simulink model "FullEKF_2007a"  (Simulink 6.6)
settings: Solver=FixedStepDiscrete  StartTime=0.0  StopTime=300  FixedStep=0.01  RelTol=1e-3
values from neighbouring files (symbols this model uses):
  initP = diag([1e-3 1e-3 1e-3 1e-6 1e-6 1e-6 1 1 1 5e-6 5e-6 5e-6 1e-8 1e-8 1e-8])    [FullEKF_init.m.m]
undefined symbols (not defined in the file or in its folder): DiscIntNeverNeededParam, gcbh, hwbcalib_subsystem
libraries: simulink x6, dspmtrx3 x4, dspinverses x1
(part 6 of 7)

== system FullEKF_2007a/INS/Attitude update/Stage2/Subsystem/a23 ==
  quat : Inport  OutDataType=fixdt(1,16,0)  OutScaling=[]  Interpolate=off  mask(Inport (HW)){maskPort=1, PortWidth=0, BusOuputAsStruct=0, signalName=<, Unit=, lowerRange=, upperRange=, InitOut=, latch=Latched}
      mask prompts: maskPort "Mask Port"; PortWidth "Dimensions (-1 for dynamic):"; BusOuputAsStruct "Output as Non-Virtual:"; signalName "Signal Name"; lowerRange "Lower Range"; upperRange "Upper Range"; InitOut "Software Initial Output"; latch "DEOS Consumed Type"
      mask init:
      | %hwbcalib_inport(gcbh,'done');
      settings: CopyFcn=hwbcalib_copyfcn(gcbh);  UndoDeleteFcn=hwbcalib_inport(gcbh,'undodelete');  ModelCloseFcn=set_param(gcbh,'DeleteFcn','');  OpenFcn=hwbcalib_inport(gcbh,0);  PreDeleteFcn=hwbcalib_inport(gcbh,'delete');
      mask Help: file:///../../../Inport.html
      mask StyleString: edit,edit,edit,edit,edit,edit,edit,edit,popup(Latched|Not Latched)
      mask Display:
      | text(4,8,['quat   [' maskPort ']'],'Horizontal','left','Vertical','middle')
      | plot([0 50-10],[0 0]);
      | plot([0 0],[0 16]);
      | plot([0 50-10],[16 16]);
      | plot([50-10 50],[16 8]);
      | plot([50-10 50],[0 8]);
  BorderBottom : Subsystem
      settings: AttributesFormatString="* HONEYWELL PROPRIETARY AND CONFIDENTIAL * Copyright (c) 1996-2011 Honeywell International Inc. * Unpublished Work.  All rights reserved. *"
      mask Type: Border (HW)
      mask Description: Border
  BorderLeft : Subsystem
      mask Type: Border (HW)
      mask Description: Border
  BorderRight : Subsystem
      mask Type: Border (HW)
      mask Description: Border
  BorderTop : Subsystem
      mask Type: Border (HW)
      mask Description: Border
  Subsystem Revision : Subsystem  mask(Subsystem Revision (HW)){trace=}
      mask prompts: trace "Trace Tag:"
      settings: CopyFcn=hwbcalib_copyfcn(gcbh);  OpenFcn=hwbcalib_subrevision(gcbh,0);
      mask Help: file:///../../../Subsystem_Revision.html
      mask Display: disp('Program: \nCPU/Process: /D:\nDLL: tgen\nFilename: INS_ham_napokusy.mdl\nSubsystem: INS/Attitude update/Stage1/quatToDcm/a23\n\nHAM Library Version: 6.5.0\nRevision: -\nDate: 07-Dec-2011 at 09:52:57\nModel Update Rate: 100 Hz\n[ode3]\nTrace Tag: \n\nPage: 18 of 53, Parent Page: 12')
  deMux : Subsystem  mask(Demux (HW)){num=4}
      mask prompts: num "Number of Outputs"
      mask init:
      | %hwbcalib_doDoneCallback('hwbcalib_demux',gcbh,99);
      settings: CopyFcn=hwbcalib_copyfcn(gcbh);  OpenFcn=hwbcalib_demux(gcbh,0);
      mask Help: file:///../../../De-Multiplexer.html
  gain : Subsystem  mask(Gain (HW)){gain=2, Ts=1/100}
      mask prompts: Ts "Sample Time"
      mask init:
      | %hwbcalib_doDoneCallback('hwbcalib_gain',gcbh,99);
      settings: CopyFcn=hwbcalib_copyfcn(gcbh);  OpenFcn=hwbcalib_gain(gcbh,0);
      mask Help: file:///../../../Gain.html
      mask Display: disp('k=2')
  product : Subsystem  mask(Product (HW)){num=2}
      mask prompts: num "Numer of Inputs"
      mask init:
      | %hwbcalib_doDoneCallback('hwbcalib_product',gcbh,99);
      settings: CopyFcn=hwbcalib_copyfcn(gcbh);  OpenFcn=hwbcalib_product(gcbh,0);
      mask Help: file:///../../../Product.html
      mask Display: disp('X')
  product1 : Subsystem  mask(Product (HW)){num=2}
      mask prompts: num "Numer of Inputs"
      mask init:
      | %hwbcalib_doDoneCallback('hwbcalib_product',gcbh,99);
      settings: CopyFcn=hwbcalib_copyfcn(gcbh);  OpenFcn=hwbcalib_product(gcbh,0);
      mask Help: file:///../../../Product.html
      mask Display: disp('X')
  sum : Subsystem  mask(Sum (HW)){signs=++}
      mask prompts: signs "String of Signs"
      mask init:
      | %hwbcalib_doDoneCallback('hwbcalib_sum',gcbh,99);
      settings: CopyFcn=hwbcalib_copyfcn(gcbh);  OpenFcn=hwbcalib_sum(gcbh,0);
      mask Help: file:///../../../Summation.html
      mask Display:
      | text(0.2, (20*(2-1)+11)/40, '+');
      | text(0.2, (20*(1-1)+11)/40, '+');
  a23 : Outport  OutDataType=fixdt(1,16,0)  OutScaling=[]  mask(Outport (HW)){maskPort=1, PortWidth=0, lowerRange=, upperRange=, signalName=<, Unit=}
      mask prompts: maskPort "Mask Port"; PortWidth "Dimensions (-1 for dynamic):"; lowerRange "Lower Range"; upperRange "Upper Range"; signalName "Signal Name"; Unit "Units"
      mask init:
      | %hwbcalib_outport(gcbh,'done');
      settings: CopyFcn=hwbcalib_copyfcn(gcbh);  UndoDeleteFcn=hwbcalib_outport(gcbh,'undodelete');  ModelCloseFcn=set_param(gcbh,'DeleteFcn','');  OpenFcn=hwbcalib_outport(gcbh,0);  PreDeleteFcn=hwbcalib_outport(gcbh,'delete');
      mask Help: file:///../../../Outport.html
      mask Display:
      | text(50-4,8,['a23   [' maskPort ']'],'Horizontal','right','Vertical','middle')
      | plot([10 50],[0 0]);
      | plot([50-1 50-1],[0 16]);
      | plot([10 50],[16 16]);
      | plot([0 10],[8 16]);
      | plot([0 10],[8 0]);
  wires:
  quat/1 -> deMux/1(Dmx)
  product/1(1000) -> sum/1(1)
  product1/1(1000) -> sum/2(2)
  sum/1(1000) -> gain/1(1)
  gain/1(2) -> a23/1
  deMux/1(1) -> product/1(1)
  deMux/2(2) -> product/2(2)
  deMux/3(3) -> product1/1(1)
  deMux/4(4) -> product1/2(2)

== system FullEKF_2007a/INS/Attitude update/Stage2/Subsystem/a31 ==
  quat : Inport  OutDataType=fixdt(1,16,0)  OutScaling=[]  Interpolate=off  mask(Inport (HW)){maskPort=1, PortWidth=0, BusOuputAsStruct=0, signalName=<, Unit=, lowerRange=, upperRange=, InitOut=, latch=Latched}
      mask prompts: maskPort "Mask Port"; PortWidth "Dimensions (-1 for dynamic):"; BusOuputAsStruct "Output as Non-Virtual:"; signalName "Signal Name"; lowerRange "Lower Range"; upperRange "Upper Range"; InitOut "Software Initial Output"; latch "DEOS Consumed Type"
      mask init:
      | %hwbcalib_inport(gcbh,'done');
      settings: CopyFcn=hwbcalib_copyfcn(gcbh);  UndoDeleteFcn=hwbcalib_inport(gcbh,'undodelete');  ModelCloseFcn=set_param(gcbh,'DeleteFcn','');  OpenFcn=hwbcalib_inport(gcbh,0);  PreDeleteFcn=hwbcalib_inport(gcbh,'delete');
      mask Help: file:///../../../Inport.html
      mask StyleString: edit,edit,edit,edit,edit,edit,edit,edit,popup(Latched|Not Latched)
      mask Display:
      | text(4,8,['quat   [' maskPort ']'],'Horizontal','left','Vertical','middle')
      | plot([0 50-10],[0 0]);
      | plot([0 0],[0 16]);
      | plot([0 50-10],[16 16]);
      | plot([50-10 50],[16 8]);
      | plot([50-10 50],[0 8]);
  BorderBottom : Subsystem
      settings: AttributesFormatString="* HONEYWELL PROPRIETARY AND CONFIDENTIAL * Copyright (c) 1996-2011 Honeywell International Inc. * Unpublished Work.  All rights reserved. *"
      mask Type: Border (HW)
      mask Description: Border
  BorderLeft : Subsystem
      mask Type: Border (HW)
      mask Description: Border
  BorderRight : Subsystem
      mask Type: Border (HW)
      mask Description: Border
  BorderTop : Subsystem
      mask Type: Border (HW)
      mask Description: Border
  Subsystem Revision : Subsystem  mask(Subsystem Revision (HW)){trace=}
      mask prompts: trace "Trace Tag:"
      settings: CopyFcn=hwbcalib_copyfcn(gcbh);  OpenFcn=hwbcalib_subrevision(gcbh,0);
      mask Help: file:///../../../Subsystem_Revision.html
      mask Display: disp('Program: \nCPU/Process: /D:\nDLL: tgen\nFilename: INS_ham_napokusy.mdl\nSubsystem: INS/Attitude update/Stage1/quatToDcm/a31\n\nHAM Library Version: 6.5.0\nRevision: -\nDate: 07-Dec-2011 at 09:52:57\nModel Update Rate: 100 Hz\n[ode3]\nTrace Tag: \n\nPage: 19 of 53, Parent Page: 12')
  deMux : Subsystem  mask(Demux (HW)){num=4}
      mask prompts: num "Number of Outputs"
      mask init:
      | %hwbcalib_doDoneCallback('hwbcalib_demux',gcbh,99);
      settings: CopyFcn=hwbcalib_copyfcn(gcbh);  OpenFcn=hwbcalib_demux(gcbh,0);
      mask Help: file:///../../../De-Multiplexer.html
  gain : Subsystem  mask(Gain (HW)){gain=2, Ts=1/100}
      mask prompts: Ts "Sample Time"
      mask init:
      | %hwbcalib_doDoneCallback('hwbcalib_gain',gcbh,99);
      settings: CopyFcn=hwbcalib_copyfcn(gcbh);  OpenFcn=hwbcalib_gain(gcbh,0);
      mask Help: file:///../../../Gain.html
      mask Display: disp('k=2')
  product : Subsystem  mask(Product (HW)){num=2}
      mask prompts: num "Numer of Inputs"
      mask init:
      | %hwbcalib_doDoneCallback('hwbcalib_product',gcbh,99);
      settings: CopyFcn=hwbcalib_copyfcn(gcbh);  OpenFcn=hwbcalib_product(gcbh,0);
      mask Help: file:///../../../Product.html
      mask Display: disp('X')
  product1 : Subsystem  mask(Product (HW)){num=2}
      mask prompts: num "Numer of Inputs"
      mask init:
      | %hwbcalib_doDoneCallback('hwbcalib_product',gcbh,99);
      settings: CopyFcn=hwbcalib_copyfcn(gcbh);  OpenFcn=hwbcalib_product(gcbh,0);
      mask Help: file:///../../../Product.html
      mask Display: disp('X')
  sum : Subsystem  mask(Sum (HW)){signs=++}
      mask prompts: signs "String of Signs"
      mask init:
      | %hwbcalib_doDoneCallback('hwbcalib_sum',gcbh,99);
      settings: CopyFcn=hwbcalib_copyfcn(gcbh);  OpenFcn=hwbcalib_sum(gcbh,0);
      mask Help: file:///../../../Summation.html
      mask Display:
      | text(0.2, (20*(2-1)+11)/40, '+');
      | text(0.2, (20*(1-1)+11)/40, '+');
  a31 : Outport  OutDataType=fixdt(1,16,0)  OutScaling=[]  mask(Outport (HW)){maskPort=1, PortWidth=0, lowerRange=, upperRange=, signalName=<, Unit=}
      mask prompts: maskPort "Mask Port"; PortWidth "Dimensions (-1 for dynamic):"; lowerRange "Lower Range"; upperRange "Upper Range"; signalName "Signal Name"; Unit "Units"
      mask init:
      | %hwbcalib_outport(gcbh,'done');
      settings: CopyFcn=hwbcalib_copyfcn(gcbh);  UndoDeleteFcn=hwbcalib_outport(gcbh,'undodelete');  ModelCloseFcn=set_param(gcbh,'DeleteFcn','');  OpenFcn=hwbcalib_outport(gcbh,0);  PreDeleteFcn=hwbcalib_outport(gcbh,'delete');
      mask Help: file:///../../../Outport.html
      mask Display:
      | text(50-4,8,['a31   [' maskPort ']'],'Horizontal','right','Vertical','middle')
      | plot([10 50],[0 0]);
      | plot([50-1 50-1],[0 16]);
      | plot([10 50],[16 16]);
      | plot([0 10],[8 16]);
      | plot([0 10],[8 0]);
  wires:
  quat/1 -> deMux/1(Dmx)
  product/1(1000) -> sum/1(1)
  product1/1(1000) -> sum/2(2)
  sum/1(1000) -> gain/1(1)
  gain/1(2) -> a31/1
  deMux/1(1) -> product/1(1)
  deMux/3(3) -> product/2(2)
  deMux/2(2) -> product1/1(1)
  deMux/4(4) -> product1/2(2)

== system FullEKF_2007a/INS/Attitude update/Stage2/Subsystem/a32 ==
  quat : Inport  OutDataType=fixdt(1,16,0)  OutScaling=[]  Interpolate=off  mask(Inport (HW)){maskPort=1, PortWidth=0, BusOuputAsStruct=0, signalName=<, Unit=, lowerRange=, upperRange=, InitOut=, latch=Latched}
      mask prompts: maskPort "Mask Port"; PortWidth "Dimensions (-1 for dynamic):"; BusOuputAsStruct "Output as Non-Virtual:"; signalName "Signal Name"; lowerRange "Lower Range"; upperRange "Upper Range"; InitOut "Software Initial Output"; latch "DEOS Consumed Type"
      mask init:
      | %hwbcalib_inport(gcbh,'done');
      settings: CopyFcn=hwbcalib_copyfcn(gcbh);  UndoDeleteFcn=hwbcalib_inport(gcbh,'undodelete');  ModelCloseFcn=set_param(gcbh,'DeleteFcn','');  OpenFcn=hwbcalib_inport(gcbh,0);  PreDeleteFcn=hwbcalib_inport(gcbh,'delete');
      mask Help: file:///../../../Inport.html
      mask StyleString: edit,edit,edit,edit,edit,edit,edit,edit,popup(Latched|Not Latched)
      mask Display:
      | text(4,8,['quat   [' maskPort ']'],'Horizontal','left','Vertical','middle')
      | plot([0 50-10],[0 0]);
      | plot([0 0],[0 16]);
      | plot([0 50-10],[16 16]);
      | plot([50-10 50],[16 8]);
      | plot([50-10 50],[0 8]);
  BorderBottom : Subsystem
      settings: AttributesFormatString="* HONEYWELL PROPRIETARY AND CONFIDENTIAL * Copyright (c) 1996-2011 Honeywell International Inc. * Unpublished Work.  All rights reserved. *"
      mask Type: Border (HW)
      mask Description: Border
  BorderLeft : Subsystem
      mask Type: Border (HW)
      mask Description: Border
  BorderRight : Subsystem
      mask Type: Border (HW)
      mask Description: Border
  BorderTop : Subsystem
      mask Type: Border (HW)
      mask Description: Border
  Subsystem Revision : Subsystem  mask(Subsystem Revision (HW)){trace=}
      mask prompts: trace "Trace Tag:"
      settings: CopyFcn=hwbcalib_copyfcn(gcbh);  OpenFcn=hwbcalib_subrevision(gcbh,0);
      mask Help: file:///../../../Subsystem_Revision.html
      mask Display: disp('Program: \nCPU/Process: /D:\nDLL: tgen\nFilename: INS_ham_napokusy.mdl\nSubsystem: INS/Attitude update/Stage1/quatToDcm/a32\n\nHAM Library Version: 6.5.0\nRevision: -\nDate: 07-Dec-2011 at 09:52:57\nModel Update Rate: 100 Hz\n[ode3]\nTrace Tag: \n\nPage: 20 of 53, Parent Page: 12')
  deMux : Subsystem  mask(Demux (HW)){num=4}
      mask prompts: num "Number of Outputs"
      mask init:
      | %hwbcalib_doDoneCallback('hwbcalib_demux',gcbh,99);
      settings: CopyFcn=hwbcalib_copyfcn(gcbh);  OpenFcn=hwbcalib_demux(gcbh,0);
      mask Help: file:///../../../De-Multiplexer.html
  gain : Subsystem  mask(Gain (HW)){gain=2, Ts=1/100}
      mask prompts: Ts "Sample Time"
      mask init:
      | %hwbcalib_doDoneCallback('hwbcalib_gain',gcbh,99);
      settings: CopyFcn=hwbcalib_copyfcn(gcbh);  OpenFcn=hwbcalib_gain(gcbh,0);
      mask Help: file:///../../../Gain.html
      mask Display: disp('k=2')
  product : Subsystem  mask(Product (HW)){num=2}
      mask prompts: num "Numer of Inputs"
      mask init:
      | %hwbcalib_doDoneCallback('hwbcalib_product',gcbh,99);
      settings: CopyFcn=hwbcalib_copyfcn(gcbh);  OpenFcn=hwbcalib_product(gcbh,0);
      mask Help: file:///../../../Product.html
      mask Display: disp('X')
  product1 : Subsystem  mask(Product (HW)){num=2}
      mask prompts: num "Numer of Inputs"
      mask init:
      | %hwbcalib_doDoneCallback('hwbcalib_product',gcbh,99);
      settings: CopyFcn=hwbcalib_copyfcn(gcbh);  OpenFcn=hwbcalib_product(gcbh,0);
      mask Help: file:///../../../Product.html
      mask Display: disp('X')
  sum : Subsystem  mask(Sum (HW)){signs=-+}
      mask prompts: signs "String of Signs"
      mask init:
      | %hwbcalib_doDoneCallback('hwbcalib_sum',gcbh,99);
      settings: CopyFcn=hwbcalib_copyfcn(gcbh);  OpenFcn=hwbcalib_sum(gcbh,0);
      mask Help: file:///../../../Summation.html
      mask Display:
      | text(0.2, (20*(2-1)+11)/40, '-');
      | text(0.2, (20*(1-1)+11)/40, '+');
  a32 : Outport  OutDataType=fixdt(1,16,0)  OutScaling=[]  mask(Outport (HW)){maskPort=1, PortWidth=0, lowerRange=, upperRange=, signalName=<, Unit=}
      mask prompts: maskPort "Mask Port"; PortWidth "Dimensions (-1 for dynamic):"; lowerRange "Lower Range"; upperRange "Upper Range"; signalName "Signal Name"; Unit "Units"
      mask init:
      | %hwbcalib_outport(gcbh,'done');
      settings: CopyFcn=hwbcalib_copyfcn(gcbh);  UndoDeleteFcn=hwbcalib_outport(gcbh,'undodelete');  ModelCloseFcn=set_param(gcbh,'DeleteFcn','');  OpenFcn=hwbcalib_outport(gcbh,0);  PreDeleteFcn=hwbcalib_outport(gcbh,'delete');
      mask Help: file:///../../../Outport.html
      mask Display:
      | text(50-4,8,['a32   [' maskPort ']'],'Horizontal','right','Vertical','middle')
      | plot([10 50],[0 0]);
      | plot([50-1 50-1],[0 16]);
      | plot([10 50],[16 16]);
      | plot([0 10],[8 16]);
      | plot([0 10],[8 0]);
  wires:
  quat/1 -> deMux/1(Dmx)
  product/1(1000) -> sum/1(1)
  product1/1(1000) -> sum/2(2)
  sum/1(1000) -> gain/1(1)
  gain/1(2) -> a32/1
  deMux/1(1) -> product/1(1)
  deMux/2(2) -> product/2(2)
  deMux/3(3) -> product1/1(1)
  deMux/4(4) -> product1/2(2)

== system FullEKF_2007a/INS/Attitude update/Stage2/Subsystem/a33 ==
  quat : Inport  OutDataType=fixdt(1,16,0)  OutScaling=[]  Interpolate=off  mask(Inport (HW)){maskPort=1, PortWidth=0, BusOuputAsStruct=0, signalName=<, Unit=, lowerRange=, upperRange=, InitOut=, latch=Latched}
      mask prompts: maskPort "Mask Port"; PortWidth "Dimensions (-1 for dynamic):"; BusOuputAsStruct "Output as Non-Virtual:"; signalName "Signal Name"; lowerRange "Lower Range"; upperRange "Upper Range"; InitOut "Software Initial Output"; latch "DEOS Consumed Type"
      mask init:
      | %hwbcalib_inport(gcbh,'done');
      settings: CopyFcn=hwbcalib_copyfcn(gcbh);  UndoDeleteFcn=hwbcalib_inport(gcbh,'undodelete');  ModelCloseFcn=set_param(gcbh,'DeleteFcn','');  OpenFcn=hwbcalib_inport(gcbh,0);  PreDeleteFcn=hwbcalib_inport(gcbh,'delete');
      mask Help: file:///../../../Inport.html
      mask StyleString: edit,edit,edit,edit,edit,edit,edit,edit,popup(Latched|Not Latched)
      mask Display:
      | text(4,8,['quat   [' maskPort ']'],'Horizontal','left','Vertical','middle')
      | plot([0 50-10],[0 0]);
      | plot([0 0],[0 16]);
      | plot([0 50-10],[16 16]);
      | plot([50-10 50],[16 8]);
      | plot([50-10 50],[0 8]);
  BorderBottom : Subsystem
      settings: AttributesFormatString="* HONEYWELL PROPRIETARY AND CONFIDENTIAL * Copyright (c) 1996-2011 Honeywell International Inc. * Unpublished Work.  All rights reserved. *"
      mask Type: Border (HW)
      mask Description: Border
  BorderLeft : Subsystem
      mask Type: Border (HW)
      mask Description: Border
  BorderRight : Subsystem
      mask Type: Border (HW)
      mask Description: Border
  BorderTop : Subsystem
      mask Type: Border (HW)
      mask Description: Border
  Subsystem Revision : Subsystem  mask(Subsystem Revision (HW)){trace=}
      mask prompts: trace "Trace Tag:"
      settings: CopyFcn=hwbcalib_copyfcn(gcbh);  OpenFcn=hwbcalib_subrevision(gcbh,0);
      mask Help: file:///../../../Subsystem_Revision.html
      mask Display: disp('Program: \nCPU/Process: /D:\nDLL: tgen\nFilename: INS_ham_napokusy.mdl\nSubsystem: INS/Attitude update/Stage1/quatToDcm/a33\n\nHAM Library Version: 6.5.0\nRevision: -\nDate: 07-Dec-2011 at 09:52:57\nModel Update Rate: 100 Hz\n[ode3]\nTrace Tag: \n\nPage: 21 of 53, Parent Page: 12')
  deMux : Subsystem  mask(Demux (HW)){num=4}
      mask prompts: num "Number of Outputs"
      mask init:
      | %hwbcalib_doDoneCallback('hwbcalib_demux',gcbh,99);
      settings: CopyFcn=hwbcalib_copyfcn(gcbh);  OpenFcn=hwbcalib_demux(gcbh,0);
      mask Help: file:///../../../De-Multiplexer.html
  product : Subsystem  mask(Product (HW)){num=2}
      mask prompts: num "Numer of Inputs"
      mask init:
      | %hwbcalib_doDoneCallback('hwbcalib_product',gcbh,99);
      settings: CopyFcn=hwbcalib_copyfcn(gcbh);  OpenFcn=hwbcalib_product(gcbh,0);
      mask Help: file:///../../../Product.html
      mask Display: disp('X')
  product1 : Subsystem  mask(Product (HW)){num=2}
      mask prompts: num "Numer of Inputs"
      mask init:
      | %hwbcalib_doDoneCallback('hwbcalib_product',gcbh,99);
      settings: CopyFcn=hwbcalib_copyfcn(gcbh);  OpenFcn=hwbcalib_product(gcbh,0);
      mask Help: file:///../../../Product.html
      mask Display: disp('X')
  product2 : Subsystem  mask(Product (HW)){num=2}
      mask prompts: num "Numer of Inputs"
      mask init:
      | %hwbcalib_doDoneCallback('hwbcalib_product',gcbh,99);
      settings: CopyFcn=hwbcalib_copyfcn(gcbh);  OpenFcn=hwbcalib_product(gcbh,0);
      mask Help: file:///../../../Product.html
      mask Display: disp('X')
  product3 : Subsystem  mask(Product (HW)){num=2}
      mask prompts: num "Numer of Inputs"
      mask init:
      | %hwbcalib_doDoneCallback('hwbcalib_product',gcbh,99);
      settings: CopyFcn=hwbcalib_copyfcn(gcbh);  OpenFcn=hwbcalib_product(gcbh,0);
      mask Help: file:///../../../Product.html
      mask Display: disp('X')
  sum : Subsystem  mask(Sum (HW)){signs=+--+}
      mask prompts: signs "String of Signs"
      mask init:
      | %hwbcalib_doDoneCallback('hwbcalib_sum',gcbh,99);
      settings: CopyFcn=hwbcalib_copyfcn(gcbh);  OpenFcn=hwbcalib_sum(gcbh,0);
      mask Help: file:///../../../Summation.html
      mask Display:
      | text(0.2, (20*(4-1)+11)/80, '+');
      | text(0.2, (20*(3-1)+11)/80, '-');
      | text(0.2, (20*(2-1)+11)/80, '-');
      | text(0.2, (20*(1-1)+11)/80, '+');
  a33 : Outport  OutDataType=fixdt(1,16,0)  OutScaling=[]  mask(Outport (HW)){maskPort=1, PortWidth=0, lowerRange=, upperRange=, signalName=<, Unit=}
      mask prompts: maskPort "Mask Port"; PortWidth "Dimensions (-1 for dynamic):"; lowerRange "Lower Range"; upperRange "Upper Range"; signalName "Signal Name"; Unit "Units"
      mask init:
      | %hwbcalib_outport(gcbh,'done');
      settings: CopyFcn=hwbcalib_copyfcn(gcbh);  UndoDeleteFcn=hwbcalib_outport(gcbh,'undodelete');  ModelCloseFcn=set_param(gcbh,'DeleteFcn','');  OpenFcn=hwbcalib_outport(gcbh,0);  PreDeleteFcn=hwbcalib_outport(gcbh,'delete');
      mask Help: file:///../../../Outport.html
      mask Display:
      | text(50-4,8,['a33   [' maskPort ']'],'Horizontal','right','Vertical','middle')
      | plot([10 50],[0 0]);
      | plot([50-1 50-1],[0 16]);
      | plot([10 50],[16 16]);
      | plot([0 10],[8 16]);
      | plot([0 10],[8 0]);
  wires:
  quat/1 -> deMux/1(Dmx)
  sum/1(1000) -> a33/1
  deMux/1(1) -> product/2(2), product/1(1)
  deMux/2(2) -> product1/1(1), product1/2(2)
  deMux/3(3) -> product2/1(1), product2/2(2)
  deMux/4(4) -> product3/2(2), product3/1(1)
  product/1(1000) -> sum/1(1)
  product1/1(1000) -> sum/2(2)
  product2/1(1000) -> sum/3(3)
  product3/1(1000) -> sum/4(4)

== system FullEKF_2007a/INS/Attitude update/Stage2/Subsystem/quat normalize ==
  q : Inport  OutDataType=fixdt(1,16,0)  OutScaling=[]
  Demux : Demux
  Mux : Mux
  Product{,1..3} (4 alike) : Product  Inputs=*/  OutDataType=fixdt(1,16,0)  OutScaling=[]
  qat modulus : Subsystem
  normal(q) : Outport  OutDataType=fixdt(1,16,0)  OutScaling=[]
  wires:
  Product3/1 -> Mux/4
  Product2/1 -> Mux/3
  Product1/1 -> Mux/2
  Product/1 -> Mux/1
  qat modulus/1(|q|) -> Product3/2, Product2/2, Product/2, Product1/2
  q/1 -> Demux/1, qat modulus/1(q)
  Mux/1 -> normal(q)/1
  Demux/1 -> Product/1
  Demux/2 -> Product1/1
  Demux/3 -> Product2/1
  Demux/4 -> Product3/1

== system FullEKF_2007a/INS/Attitude update/Stage2/eulerToQuat/a1 ==
  attInitCon : Inport  OutDataType=fixdt(1,16,0)  OutScaling=[]
  Demux : Demux  Outputs=3
  Gain : Gain  Gain=0.5  ParameterDataType=fixdt(1,16,0)  ParameterScaling=[]  OutDataType=fixdt(1,16,0)  OutScaling=[]  SampleTime=0.01
  Gain1 : Gain  Gain=0.5  ParameterDataType=fixdt(1,16,0)  ParameterScaling=[]  OutDataType=fixdt(1,16,0)  OutScaling=[]  SampleTime=0.01
  Gain2 : Gain  Gain=0.5  ParameterDataType=fixdt(1,16,0)  ParameterScaling=[]  OutDataType=fixdt(1,16,0)  OutScaling=[]  SampleTime=0.01
  Product : Product  Inputs=3  OutDataType=fixdt(1,16,0)  OutScaling=[]  SampleTime=0.01  RndMeth=Zero
  Product1 : Product  Inputs=3  OutDataType=fixdt(1,16,0)  OutScaling=[]  SampleTime=0.01  RndMeth=Zero
  Sum : Sum  Inputs=|++  OutDataType=fixdt(1,16,0)  OutScaling=[]
  Trigonometric Function : Trigonometry  Operator=cos  SampleTime=0.01
  Trigonometric Function1 : Trigonometry  Operator=cos  SampleTime=0.01
  Trigonometric Function2 : Trigonometry  Operator=cos  SampleTime=0.01
  Trigonometric Function3 : Trigonometry
  Trigonometric Function4 : Trigonometry
  a1 : Outport  OutDataType=fixdt(1,16,0)  OutScaling=[]
  wires:
  attInitCon/1 -> Demux/1
  Demux/1 -> Gain2/1
  Demux/2 -> Gain/1
  Demux/3 -> Gain1/1
  Gain2/1 -> Trigonometric Function/1, Trigonometric Function3/1
  Gain/1 -> Trigonometric Function1/1, Trigonometric Function4/1
  Gain1/1 -> Trigonometric Function2/1
  Trigonometric Function/1 -> Product/1
  Trigonometric Function1/1 -> Product/2
  Trigonometric Function2/1 -> Product/3, Product1/1
  Product/1 -> Sum/1
  Sum/1 -> a1/1
  Trigonometric Function4/1 -> Product1/3
  Trigonometric Function3/1 -> Product1/2
  Product1/1 -> Sum/2

== system FullEKF_2007a/INS/Attitude update/Stage2/eulerToQuat/a2 ==
  attInitCon : Inport  OutDataType=fixdt(1,16,0)  OutScaling=[]
  Demux : Demux  Outputs=3
  Gain : Gain  Gain=0.5  ParameterDataType=fixdt(1,16,0)  ParameterScaling=[]  OutDataType=fixdt(1,16,0)  OutScaling=[]  SampleTime=0.01
  Gain1 : Gain  Gain=0.5  ParameterDataType=fixdt(1,16,0)  ParameterScaling=[]  OutDataType=fixdt(1,16,0)  OutScaling=[]  SampleTime=0.01
  Gain2 : Gain  Gain=0.5  ParameterDataType=fixdt(1,16,0)  ParameterScaling=[]  OutDataType=fixdt(1,16,0)  OutScaling=[]  SampleTime=0.01
  Product : Product  Inputs=3  OutDataType=fixdt(1,16,0)  OutScaling=[]  SampleTime=0.01  RndMeth=Zero
  Product1 : Product  Inputs=3  OutDataType=fixdt(1,16,0)  OutScaling=[]  SampleTime=0.01  RndMeth=Zero
  Sum : Sum  Inputs=|+-  OutDataType=fixdt(1,16,0)  OutScaling=[]  SampleTime=0.01
  Trigonometric Function : Trigonometry  SampleTime=0.01
  Trigonometric Function1 : Trigonometry  Operator=cos  SampleTime=0.01
  Trigonometric Function2 : Trigonometry  Operator=cos  SampleTime=0.01
  Trigonometric Function3 : Trigonometry
  Trigonometric Function4 : Trigonometry
  Trigonometric Function5 : Trigonometry  Operator=cos  SampleTime=0.01
  a2 : Outport  OutDataType=fixdt(1,16,0)  OutScaling=[]
  wires:
  attInitCon/1 -> Demux/1
  Demux/1 -> Gain2/1
  Demux/2 -> Gain/1
  Demux/3 -> Gain1/1
  Gain2/1 -> Trigonometric Function/1, Trigonometric Function3/1, Trigonometric Function5/1
  Gain/1 -> Trigonometric Function1/1
  Gain1/1 -> Trigonometric Function2/1, Trigonometric Function4/1
  Trigonometric Function/1 -> Product/1
  Trigonometric Function1/1 -> Product/2
  Trigonometric Function2/1 -> Product/3
  Product/1 -> Sum/1
  Sum/1 -> a2/1
  Product1/1 -> Sum/2
  Trigonometric Function5/1 -> Product1/3
  Trigonometric Function4/1 -> Product1/2
  Trigonometric Function3/1 -> Product1/1

== system FullEKF_2007a/INS/Attitude update/Stage2/eulerToQuat/a3 ==
  attInitCon : Inport  OutDataType=fixdt(1,16,0)  OutScaling=[]
  Demux : Demux  Outputs=3
  Gain : Gain  Gain=0.5  ParameterDataType=fixdt(1,16,0)  ParameterScaling=[]  OutDataType=fixdt(1,16,0)  OutScaling=[]  SampleTime=0.01
  Gain1 : Gain  Gain=0.5  ParameterDataType=fixdt(1,16,0)  ParameterScaling=[]  OutDataType=fixdt(1,16,0)  OutScaling=[]  SampleTime=0.01
  Gain2 : Gain  Gain=0.5  ParameterDataType=fixdt(1,16,0)  ParameterScaling=[]  OutDataType=fixdt(1,16,0)  OutScaling=[]  SampleTime=0.01
  Product : Product  Inputs=3  OutDataType=fixdt(1,16,0)  OutScaling=[]  SampleTime=0.01  RndMeth=Zero
  Product1 : Product  Inputs=3  OutDataType=fixdt(1,16,0)  OutScaling=[]  SampleTime=0.01  RndMeth=Zero
  Sum : Sum  OutDataType=fixdt(1,16,0)  OutScaling=[]  SampleTime=0.01
  Trigonometric Function : Trigonometry  Operator=cos  SampleTime=0.01
  Trigonometric Function1 : Trigonometry  SampleTime=0.01
  Trigonometric Function3 : Trigonometry  Operator=cos  SampleTime=0.01
  Trigonometric Function4 : Trigonometry  Operator=cos  SampleTime=0.01
  Trigonometric Function5 : Trigonometry
  a3 : Outport  OutDataType=fixdt(1,16,0)  OutScaling=[]
  wires:
  attInitCon/1 -> Demux/1
  Demux/1 -> Gain2/1
  Demux/2 -> Gain/1
  Demux/3 -> Gain1/1
  Gain2/1 -> Product1/3, Trigonometric Function/1
  Gain/1 -> Trigonometric Function1/1, Trigonometric Function4/1
  Gain1/1 -> Trigonometric Function3/1, Trigonometric Function5/1
  Trigonometric Function/1 -> Product/1
  Trigonometric Function1/1 -> Product/2
  Trigonometric Function3/1 -> Product/3
  Product/1 -> Sum/1
  Sum/1 -> a3/1
  Product1/1 -> Sum/2
  Trigonometric Function4/1 -> Product1/1
  Trigonometric Function5/1 -> Product1/2

== system FullEKF_2007a/INS/Attitude update/Stage2/eulerToQuat/a4 ==
  attInitCon : Inport  OutDataType=fixdt(1,16,0)  OutScaling=[]
  Demux : Demux  Outputs=3
  Gain : Gain  Gain=0.5  ParameterDataType=fixdt(1,16,0)  ParameterScaling=[]  OutDataType=fixdt(1,16,0)  OutScaling=[]  SampleTime=0.01
  Gain1 : Gain  Gain=0.5  ParameterDataType=fixdt(1,16,0)  ParameterScaling=[]  OutDataType=fixdt(1,16,0)  OutScaling=[]  SampleTime=0.01
  Gain2 : Gain  Gain=0.5  ParameterDataType=fixdt(1,16,0)  ParameterScaling=[]  OutDataType=fixdt(1,16,0)  OutScaling=[]  SampleTime=0.01
  Product : Product  Inputs=3  OutDataType=fixdt(1,16,0)  OutScaling=[]  SampleTime=0.01  RndMeth=Zero
  Product1 : Product  Inputs=3  OutDataType=fixdt(1,16,0)  OutScaling=[]  SampleTime=0.01  RndMeth=Zero
  Sum : Sum  Inputs=|+-  OutDataType=fixdt(1,16,0)  OutScaling=[]  SampleTime=0.01
  Trigonometric Function : Trigonometry  Operator=cos  SampleTime=0.01
  Trigonometric Function1 : Trigonometry  Operator=cos  SampleTime=0.01
  Trigonometric Function2 : Trigonometry  SampleTime=0.01
  Trigonometric Function3 : Trigonometry
  Trigonometric Function4 : Trigonometry  Operator=cos  SampleTime=0.01
  Trigonometric Function5 : Trigonometry  SampleTime=0.01
  a2 : Outport  OutDataType=fixdt(1,16,0)  OutScaling=[]
  wires:
  attInitCon/1 -> Demux/1
  Demux/1 -> Gain2/1
  Demux/2 -> Gain/1
  Demux/3 -> Gain1/1
  Gain2/1 -> Trigonometric Function/1, Trigonometric Function3/1
  Gain/1 -> Trigonometric Function1/1, Trigonometric Function5/1
  Gain1/1 -> Trigonometric Function2/1, Trigonometric Function4/1
  Trigonometric Function/1 -> Product/1
  Trigonometric Function1/1 -> Product/2
  Trigonometric Function2/1 -> Product/3
  Product/1 -> Sum/1
  Sum/1 -> a2/1
  Product1/1 -> Sum/2
  Trigonometric Function3/1 -> Product1/1
  Trigonometric Function4/1 -> Product1/2
  Trigonometric Function5/1 -> Product1/3

== system FullEKF_2007a/INS/Attitude update/Stage2/Subsystem/a11/BorderBottom ==

== system FullEKF_2007a/INS/Attitude update/Stage2/Subsystem/a11/BorderLeft ==

== system FullEKF_2007a/INS/Attitude update/Stage2/Subsystem/a11/BorderRight ==

== system FullEKF_2007a/INS/Attitude update/Stage2/Subsystem/a11/BorderTop ==

== system FullEKF_2007a/INS/Attitude update/Stage2/Subsystem/a11/Subsystem Revision ==

== system FullEKF_2007a/INS/Attitude update/Stage2/Subsystem/a11/deMux ==
  Dmx : Inport  OutDataType=fixdt(1,16,0)  OutScaling=[]
  999 : Demux
  1 : Outport  OutDataType=fixdt(1,16,0)  OutScaling=[]
  2 : Outport  Port=2  OutDataType=fixdt(1,16,0)  OutScaling=[]
  3 : Outport  Port=3  OutDataType=fixdt(1,16,0)  OutScaling=[]
  4 : Outport  Port=4  OutDataType=fixdt(1,16,0)  OutScaling=[]
  wires:
  999/1 -> 1/1
  999/2 -> 2/1
  Dmx/1 -> 999/1
  999/3 -> 3/1
  999/4 -> 4/1

== system FullEKF_2007a/INS/Attitude update/Stage2/Subsystem/a11/product ==
  1 : Inport  OutDataType=fixdt(1,16,0)  OutScaling=[]
  2 : Inport  Port=2  OutDataType=fixdt(1,16,0)  OutScaling=[]
  Product_1 : Product  OutDataType=fixdt(1,16,0)  OutScaling=[]  RndMeth=Zero  InputSameDT=on
  1000 : Outport  OutDataType=fixdt(1,16,0)  OutScaling=[]
  wires:
  Product_1/1 -> 1000/1
  1/1 -> Product_1/1
  2/1 -> Product_1/2

== system FullEKF_2007a/INS/Attitude update/Stage2/Subsystem/a11/product1 ==
  1 : Inport  OutDataType=fixdt(1,16,0)  OutScaling=[]
  2 : Inport  Port=2  OutDataType=fixdt(1,16,0)  OutScaling=[]
  Product_1 : Product  OutDataType=fixdt(1,16,0)  OutScaling=[]  RndMeth=Zero  InputSameDT=on
  1000 : Outport  OutDataType=fixdt(1,16,0)  OutScaling=[]
  wires:
  Product_1/1 -> 1000/1
  1/1 -> Product_1/1
  2/1 -> Product_1/2

== system FullEKF_2007a/INS/Attitude update/Stage2/Subsystem/a11/product2 ==
  1 : Inport  OutDataType=fixdt(1,16,0)  OutScaling=[]
  2 : Inport  Port=2  OutDataType=fixdt(1,16,0)  OutScaling=[]
  Product_1 : Product  OutDataType=fixdt(1,16,0)  OutScaling=[]  RndMeth=Zero  InputSameDT=on
  1000 : Outport  OutDataType=fixdt(1,16,0)  OutScaling=[]
  wires:
  Product_1/1 -> 1000/1
  1/1 -> Product_1/1
  2/1 -> Product_1/2

== system FullEKF_2007a/INS/Attitude update/Stage2/Subsystem/a11/product3 ==
  1 : Inport  OutDataType=fixdt(1,16,0)  OutScaling=[]
  2 : Inport  Port=2  OutDataType=fixdt(1,16,0)  OutScaling=[]
  Product_1 : Product  OutDataType=fixdt(1,16,0)  OutScaling=[]  RndMeth=Zero  InputSameDT=on
  1000 : Outport  OutDataType=fixdt(1,16,0)  OutScaling=[]
  wires:
  Product_1/1 -> 1000/1
  1/1 -> Product_1/1
  2/1 -> Product_1/2

== system FullEKF_2007a/INS/Attitude update/Stage2/Subsystem/a11/sum ==
  1 : Inport  OutDataType=fixdt(1,16,0)  OutScaling=[]
  2 : Inport  Port=2  OutDataType=fixdt(1,16,0)  OutScaling=[]
  3 : Inport  Port=3  OutDataType=fixdt(1,16,0)  OutScaling=[]
  4 : Inport  Port=4  OutDataType=fixdt(1,16,0)  OutScaling=[]
  Sum_1 : Sum  Inputs=++--  OutDataType=fixdt(1,16,0)  OutScaling=[]  RndMeth=Zero  InputSameDT=on
  1000 : Outport  OutDataType=fixdt(1,16,0)  OutScaling=[]
  wires:
  Sum_1/1 -> 1000/1
  1/1 -> Sum_1/1
  2/1 -> Sum_1/2
  3/1 -> Sum_1/3
  4/1 -> Sum_1/4

== system FullEKF_2007a/INS/Attitude update/Stage2/Subsystem/a12/BorderBottom ==

== system FullEKF_2007a/INS/Attitude update/Stage2/Subsystem/a12/BorderLeft ==

== system FullEKF_2007a/INS/Attitude update/Stage2/Subsystem/a12/BorderRight ==

== system FullEKF_2007a/INS/Attitude update/Stage2/Subsystem/a12/BorderTop ==

== system FullEKF_2007a/INS/Attitude update/Stage2/Subsystem/a12/Subsystem Revision ==

== system FullEKF_2007a/INS/Attitude update/Stage2/Subsystem/a12/deMux ==
  Dmx : Inport  OutDataType=fixdt(1,16,0)  OutScaling=[]
  999 : Demux
  1 : Outport  OutDataType=fixdt(1,16,0)  OutScaling=[]
  2 : Outport  Port=2  OutDataType=fixdt(1,16,0)  OutScaling=[]
  3 : Outport  Port=3  OutDataType=fixdt(1,16,0)  OutScaling=[]
  4 : Outport  Port=4  OutDataType=fixdt(1,16,0)  OutScaling=[]
  wires:
  999/1 -> 1/1
  999/2 -> 2/1
  Dmx/1 -> 999/1
  999/3 -> 3/1
  999/4 -> 4/1

== system FullEKF_2007a/INS/Attitude update/Stage2/Subsystem/a12/gain ==
  1 : Inport  OutDataType=fixdt(1,16,0)  OutScaling=[]
  Gain_1 : Gain  Gain=eval(gain)  ParameterDataType=fixdt(1,16,0)  ParameterScaling=[]  OutDataType=fixdt(1,16,0)  OutScaling=[]  RndMeth=Zero
  2 : Outport  OutDataType=fixdt(1,16,0)  OutScaling=[]
  wires:
  1/1 -> Gain_1/1
  Gain_1/1 -> 2/1

== system FullEKF_2007a/INS/Attitude update/Stage2/Subsystem/a12/product ==
  1 : Inport  OutDataType=fixdt(1,16,0)  OutScaling=[]
  2 : Inport  Port=2  OutDataType=fixdt(1,16,0)  OutScaling=[]
  Product_1 : Product  OutDataType=fixdt(1,16,0)  OutScaling=[]  RndMeth=Zero  InputSameDT=on
  1000 : Outport  OutDataType=fixdt(1,16,0)  OutScaling=[]
  wires:
  Product_1/1 -> 1000/1
  1/1 -> Product_1/1
  2/1 -> Product_1/2

== system FullEKF_2007a/INS/Attitude update/Stage2/Subsystem/a12/product1 ==
  1 : Inport  OutDataType=fixdt(1,16,0)  OutScaling=[]
  2 : Inport  Port=2  OutDataType=fixdt(1,16,0)  OutScaling=[]
  Product_1 : Product  OutDataType=fixdt(1,16,0)  OutScaling=[]  RndMeth=Zero  InputSameDT=on
  1000 : Outport  OutDataType=fixdt(1,16,0)  OutScaling=[]
  wires:
  Product_1/1 -> 1000/1
  1/1 -> Product_1/1
  2/1 -> Product_1/2

== system FullEKF_2007a/INS/Attitude update/Stage2/Subsystem/a12/sum ==
  1 : Inport  OutDataType=fixdt(1,16,0)  OutScaling=[]
  2 : Inport  Port=2  OutDataType=fixdt(1,16,0)  OutScaling=[]
  Sum_1 : Sum  OutDataType=fixdt(1,16,0)  OutScaling=[]  RndMeth=Zero  InputSameDT=on
  1000 : Outport  OutDataType=fixdt(1,16,0)  OutScaling=[]
  wires:
  Sum_1/1 -> 1000/1
  1/1 -> Sum_1/1
  2/1 -> Sum_1/2

== system FullEKF_2007a/INS/Attitude update/Stage2/Subsystem/a13/BorderBottom ==

== system FullEKF_2007a/INS/Attitude update/Stage2/Subsystem/a13/BorderLeft ==

== system FullEKF_2007a/INS/Attitude update/Stage2/Subsystem/a13/BorderRight ==

== system FullEKF_2007a/INS/Attitude update/Stage2/Subsystem/a13/BorderTop ==

== system FullEKF_2007a/INS/Attitude update/Stage2/Subsystem/a13/Subsystem Revision ==

== system FullEKF_2007a/INS/Attitude update/Stage2/Subsystem/a13/deMux ==
  Dmx : Inport  OutDataType=fixdt(1,16,0)  OutScaling=[]
  999 : Demux
  1 : Outport  OutDataType=fixdt(1,16,0)  OutScaling=[]
  2 : Outport  Port=2  OutDataType=fixdt(1,16,0)  OutScaling=[]
  3 : Outport  Port=3  OutDataType=fixdt(1,16,0)  OutScaling=[]
  4 : Outport  Port=4  OutDataType=fixdt(1,16,0)  OutScaling=[]
  wires:
  999/1 -> 1/1
  999/2 -> 2/1
  Dmx/1 -> 999/1
  999/3 -> 3/1
  999/4 -> 4/1

== system FullEKF_2007a/INS/Attitude update/Stage2/Subsystem/a13/gain ==
  1 : Inport  OutDataType=fixdt(1,16,0)  OutScaling=[]
  Gain_1 : Gain  Gain=eval(gain)  ParameterDataType=fixdt(1,16,0)  ParameterScaling=[]  OutDataType=fixdt(1,16,0)  OutScaling=[]  RndMeth=Zero
  2 : Outport  OutDataType=fixdt(1,16,0)  OutScaling=[]
  wires:
  1/1 -> Gain_1/1
  Gain_1/1 -> 2/1

== system FullEKF_2007a/INS/Attitude update/Stage2/Subsystem/a13/product ==
  1 : Inport  OutDataType=fixdt(1,16,0)  OutScaling=[]
  2 : Inport  Port=2  OutDataType=fixdt(1,16,0)  OutScaling=[]
  Product_1 : Product  OutDataType=fixdt(1,16,0)  OutScaling=[]  RndMeth=Zero  InputSameDT=on
  1000 : Outport  OutDataType=fixdt(1,16,0)  OutScaling=[]
  wires:
  Product_1/1 -> 1000/1
  1/1 -> Product_1/1
  2/1 -> Product_1/2

== system FullEKF_2007a/INS/Attitude update/Stage2/Subsystem/a13/product1 ==
  1 : Inport  OutDataType=fixdt(1,16,0)  OutScaling=[]
  2 : Inport  Port=2  OutDataType=fixdt(1,16,0)  OutScaling=[]
  Product_1 : Product  OutDataType=fixdt(1,16,0)  OutScaling=[]  RndMeth=Zero  InputSameDT=on
  1000 : Outport  OutDataType=fixdt(1,16,0)  OutScaling=[]
  wires:
  Product_1/1 -> 1000/1
  1/1 -> Product_1/1
  2/1 -> Product_1/2

== system FullEKF_2007a/INS/Attitude update/Stage2/Subsystem/a13/sum ==
  1 : Inport  OutDataType=fixdt(1,16,0)  OutScaling=[]
  2 : Inport  Port=2  OutDataType=fixdt(1,16,0)  OutScaling=[]
  Sum_1 : Sum  Inputs=-+  OutDataType=fixdt(1,16,0)  OutScaling=[]  RndMeth=Zero  InputSameDT=on
  1000 : Outport  OutDataType=fixdt(1,16,0)  OutScaling=[]
  wires:
  Sum_1/1 -> 1000/1
  1/1 -> Sum_1/1
  2/1 -> Sum_1/2

== system FullEKF_2007a/INS/Attitude update/Stage2/Subsystem/a21/BorderBottom ==

== system FullEKF_2007a/INS/Attitude update/Stage2/Subsystem/a21/BorderLeft ==

== system FullEKF_2007a/INS/Attitude update/Stage2/Subsystem/a21/BorderRight ==

== system FullEKF_2007a/INS/Attitude update/Stage2/Subsystem/a21/BorderTop ==

== system FullEKF_2007a/INS/Attitude update/Stage2/Subsystem/a21/Subsystem Revision ==

== system FullEKF_2007a/INS/Attitude update/Stage2/Subsystem/a21/deMux ==
  Dmx : Inport  OutDataType=fixdt(1,16,0)  OutScaling=[]
  999 : Demux
  1 : Outport  OutDataType=fixdt(1,16,0)  OutScaling=[]
  2 : Outport  Port=2  OutDataType=fixdt(1,16,0)  OutScaling=[]
  3 : Outport  Port=3  OutDataType=fixdt(1,16,0)  OutScaling=[]
  4 : Outport  Port=4  OutDataType=fixdt(1,16,0)  OutScaling=[]
  wires:
  999/1 -> 1/1
  999/2 -> 2/1
  Dmx/1 -> 999/1
  999/3 -> 3/1
  999/4 -> 4/1

== system FullEKF_2007a/INS/Attitude update/Stage2/Subsystem/a21/gain ==
  1 : Inport  OutDataType=fixdt(1,16,0)  OutScaling=[]
  Gain_1 : Gain  Gain=eval(gain)  ParameterDataType=fixdt(1,16,0)  ParameterScaling=[]  OutDataType=fixdt(1,16,0)  OutScaling=[]  RndMeth=Zero
  2 : Outport  OutDataType=fixdt(1,16,0)  OutScaling=[]
  wires:
  1/1 -> Gain_1/1
  Gain_1/1 -> 2/1

== system FullEKF_2007a/INS/Attitude update/Stage2/Subsystem/a21/product ==
  1 : Inport  OutDataType=fixdt(1,16,0)  OutScaling=[]
  2 : Inport  Port=2  OutDataType=fixdt(1,16,0)  OutScaling=[]
  Product_1 : Product  OutDataType=fixdt(1,16,0)  OutScaling=[]  RndMeth=Zero  InputSameDT=on
  1000 : Outport  OutDataType=fixdt(1,16,0)  OutScaling=[]
  wires:
  Product_1/1 -> 1000/1
  1/1 -> Product_1/1
  2/1 -> Product_1/2

== system FullEKF_2007a/INS/Attitude update/Stage2/Subsystem/a21/product1 ==
  1 : Inport  OutDataType=fixdt(1,16,0)  OutScaling=[]
  2 : Inport  Port=2  OutDataType=fixdt(1,16,0)  OutScaling=[]
  Product_1 : Product  OutDataType=fixdt(1,16,0)  OutScaling=[]  RndMeth=Zero  InputSameDT=on
  1000 : Outport  OutDataType=fixdt(1,16,0)  OutScaling=[]
  wires:
  Product_1/1 -> 1000/1
  1/1 -> Product_1/1
  2/1 -> Product_1/2

== system FullEKF_2007a/INS/Attitude update/Stage2/Subsystem/a21/sum ==
  1 : Inport  OutDataType=fixdt(1,16,0)  OutScaling=[]
  2 : Inport  Port=2  OutDataType=fixdt(1,16,0)  OutScaling=[]
  Sum_1 : Sum  Inputs=-+  OutDataType=fixdt(1,16,0)  OutScaling=[]  RndMeth=Zero  InputSameDT=on
  1000 : Outport  OutDataType=fixdt(1,16,0)  OutScaling=[]
  wires:
  Sum_1/1 -> 1000/1
  1/1 -> Sum_1/1
  2/1 -> Sum_1/2

== system FullEKF_2007a/INS/Attitude update/Stage2/Subsystem/a22/BorderBottom ==

== system FullEKF_2007a/INS/Attitude update/Stage2/Subsystem/a22/BorderLeft ==

== system FullEKF_2007a/INS/Attitude update/Stage2/Subsystem/a22/BorderRight ==

== system FullEKF_2007a/INS/Attitude update/Stage2/Subsystem/a22/BorderTop ==

== system FullEKF_2007a/INS/Attitude update/Stage2/Subsystem/a22/Subsystem Revision ==

== system FullEKF_2007a/INS/Attitude update/Stage2/Subsystem/a22/deMux ==
  Dmx : Inport  OutDataType=fixdt(1,16,0)  OutScaling=[]
  999 : Demux
  1 : Outport  OutDataType=fixdt(1,16,0)  OutScaling=[]
  2 : Outport  Port=2  OutDataType=fixdt(1,16,0)  OutScaling=[]
  3 : Outport  Port=3  OutDataType=fixdt(1,16,0)  OutScaling=[]
  4 : Outport  Port=4  OutDataType=fixdt(1,16,0)  OutScaling=[]
  wires:
  999/1 -> 1/1
  999/2 -> 2/1
  Dmx/1 -> 999/1
  999/3 -> 3/1
  999/4 -> 4/1

== system FullEKF_2007a/INS/Attitude update/Stage2/Subsystem/a22/product ==
  1 : Inport  OutDataType=fixdt(1,16,0)  OutScaling=[]
  2 : Inport  Port=2  OutDataType=fixdt(1,16,0)  OutScaling=[]
  Product_1 : Product  OutDataType=fixdt(1,16,0)  OutScaling=[]  RndMeth=Zero  InputSameDT=on
  1000 : Outport  OutDataType=fixdt(1,16,0)  OutScaling=[]
  wires:
  Product_1/1 -> 1000/1
  1/1 -> Product_1/1
  2/1 -> Product_1/2

== system FullEKF_2007a/INS/Attitude update/Stage2/Subsystem/a22/product1 ==
  1 : Inport  OutDataType=fixdt(1,16,0)  OutScaling=[]
  2 : Inport  Port=2  OutDataType=fixdt(1,16,0)  OutScaling=[]
  Product_1 : Product  OutDataType=fixdt(1,16,0)  OutScaling=[]  RndMeth=Zero  InputSameDT=on
  1000 : Outport  OutDataType=fixdt(1,16,0)  OutScaling=[]
  wires:
  Product_1/1 -> 1000/1
  1/1 -> Product_1/1
  2/1 -> Product_1/2

== system FullEKF_2007a/INS/Attitude update/Stage2/Subsystem/a22/product2 ==
  1 : Inport  OutDataType=fixdt(1,16,0)  OutScaling=[]
  2 : Inport  Port=2  OutDataType=fixdt(1,16,0)  OutScaling=[]
  Product_1 : Product  OutDataType=fixdt(1,16,0)  OutScaling=[]  RndMeth=Zero  InputSameDT=on
  1000 : Outport  OutDataType=fixdt(1,16,0)  OutScaling=[]
  wires:
  Product_1/1 -> 1000/1
  1/1 -> Product_1/1
  2/1 -> Product_1/2

== system FullEKF_2007a/INS/Attitude update/Stage2/Subsystem/a22/product3 ==
  1 : Inport  OutDataType=fixdt(1,16,0)  OutScaling=[]
  2 : Inport  Port=2  OutDataType=fixdt(1,16,0)  OutScaling=[]
  Product_1 : Product  OutDataType=fixdt(1,16,0)  OutScaling=[]  RndMeth=Zero  InputSameDT=on
  1000 : Outport  OutDataType=fixdt(1,16,0)  OutScaling=[]
  wires:
  Product_1/1 -> 1000/1
  1/1 -> Product_1/1
  2/1 -> Product_1/2

== system FullEKF_2007a/INS/Attitude update/Stage2/Subsystem/a22/sum ==
  1 : Inport  OutDataType=fixdt(1,16,0)  OutScaling=[]
  2 : Inport  Port=2  OutDataType=fixdt(1,16,0)  OutScaling=[]
  3 : Inport  Port=3  OutDataType=fixdt(1,16,0)  OutScaling=[]
  4 : Inport  Port=4  OutDataType=fixdt(1,16,0)  OutScaling=[]
  Sum_1 : Sum  Inputs=+-+-  OutDataType=fixdt(1,16,0)  OutScaling=[]  RndMeth=Zero  InputSameDT=on
  1000 : Outport  OutDataType=fixdt(1,16,0)  OutScaling=[]
  wires:
  Sum_1/1 -> 1000/1
  1/1 -> Sum_1/1
  2/1 -> Sum_1/2
  3/1 -> Sum_1/3
  4/1 -> Sum_1/4

== system FullEKF_2007a/INS/Attitude update/Stage2/Subsystem/a23/BorderBottom ==

== system FullEKF_2007a/INS/Attitude update/Stage2/Subsystem/a23/BorderLeft ==

== system FullEKF_2007a/INS/Attitude update/Stage2/Subsystem/a23/BorderRight ==

== system FullEKF_2007a/INS/Attitude update/Stage2/Subsystem/a23/BorderTop ==

== system FullEKF_2007a/INS/Attitude update/Stage2/Subsystem/a23/Subsystem Revision ==

== system FullEKF_2007a/INS/Attitude update/Stage2/Subsystem/a23/deMux ==
  Dmx : Inport  OutDataType=fixdt(1,16,0)  OutScaling=[]
  999 : Demux
  1 : Outport  OutDataType=fixdt(1,16,0)  OutScaling=[]
  2 : Outport  Port=2  OutDataType=fixdt(1,16,0)  OutScaling=[]
  3 : Outport  Port=3  OutDataType=fixdt(1,16,0)  OutScaling=[]
  4 : Outport  Port=4  OutDataType=fixdt(1,16,0)  OutScaling=[]
  wires:
  999/1 -> 1/1
  999/2 -> 2/1
  Dmx/1 -> 999/1
  999/3 -> 3/1
  999/4 -> 4/1

== system FullEKF_2007a/INS/Attitude update/Stage2/Subsystem/a23/gain ==
  1 : Inport  OutDataType=fixdt(1,16,0)  OutScaling=[]
  Gain_1 : Gain  Gain=eval(gain)  ParameterDataType=fixdt(1,16,0)  ParameterScaling=[]  OutDataType=fixdt(1,16,0)  OutScaling=[]  RndMeth=Zero
  2 : Outport  OutDataType=fixdt(1,16,0)  OutScaling=[]
  wires:
  1/1 -> Gain_1/1
  Gain_1/1 -> 2/1

== system FullEKF_2007a/INS/Attitude update/Stage2/Subsystem/a23/product ==
  1 : Inport  OutDataType=fixdt(1,16,0)  OutScaling=[]
  2 : Inport  Port=2  OutDataType=fixdt(1,16,0)  OutScaling=[]
  Product_1 : Product  OutDataType=fixdt(1,16,0)  OutScaling=[]  RndMeth=Zero  InputSameDT=on
  1000 : Outport  OutDataType=fixdt(1,16,0)  OutScaling=[]
  wires:
  Product_1/1 -> 1000/1
  1/1 -> Product_1/1
  2/1 -> Product_1/2

== system FullEKF_2007a/INS/Attitude update/Stage2/Subsystem/a23/product1 ==
  1 : Inport  OutDataType=fixdt(1,16,0)  OutScaling=[]
  2 : Inport  Port=2  OutDataType=fixdt(1,16,0)  OutScaling=[]
  Product_1 : Product  OutDataType=fixdt(1,16,0)  OutScaling=[]  RndMeth=Zero  InputSameDT=on
  1000 : Outport  OutDataType=fixdt(1,16,0)  OutScaling=[]
  wires:
  Product_1/1 -> 1000/1
  1/1 -> Product_1/1
  2/1 -> Product_1/2

== system FullEKF_2007a/INS/Attitude update/Stage2/Subsystem/a23/sum ==
  1 : Inport  OutDataType=fixdt(1,16,0)  OutScaling=[]
  2 : Inport  Port=2  OutDataType=fixdt(1,16,0)  OutScaling=[]
  Sum_1 : Sum  OutDataType=fixdt(1,16,0)  OutScaling=[]  RndMeth=Zero  InputSameDT=on
  1000 : Outport  OutDataType=fixdt(1,16,0)  OutScaling=[]
  wires:
  Sum_1/1 -> 1000/1
  1/1 -> Sum_1/1
  2/1 -> Sum_1/2

== system FullEKF_2007a/INS/Attitude update/Stage2/Subsystem/a31/BorderBottom ==

== system FullEKF_2007a/INS/Attitude update/Stage2/Subsystem/a31/BorderLeft ==

== system FullEKF_2007a/INS/Attitude update/Stage2/Subsystem/a31/BorderRight ==

== system FullEKF_2007a/INS/Attitude update/Stage2/Subsystem/a31/BorderTop ==

== system FullEKF_2007a/INS/Attitude update/Stage2/Subsystem/a31/Subsystem Revision ==

== system FullEKF_2007a/INS/Attitude update/Stage2/Subsystem/a31/deMux ==
  Dmx : Inport  OutDataType=fixdt(1,16,0)  OutScaling=[]
  999 : Demux
  1 : Outport  OutDataType=fixdt(1,16,0)  OutScaling=[]
  2 : Outport  Port=2  OutDataType=fixdt(1,16,0)  OutScaling=[]
  3 : Outport  Port=3  OutDataType=fixdt(1,16,0)  OutScaling=[]
  4 : Outport  Port=4  OutDataType=fixdt(1,16,0)  OutScaling=[]
  wires:
  999/1 -> 1/1
  999/2 -> 2/1
  Dmx/1 -> 999/1
  999/3 -> 3/1
  999/4 -> 4/1

== system FullEKF_2007a/INS/Attitude update/Stage2/Subsystem/a31/gain ==
  1 : Inport  OutDataType=fixdt(1,16,0)  OutScaling=[]
  Gain_1 : Gain  Gain=eval(gain)  ParameterDataType=fixdt(1,16,0)  ParameterScaling=[]  OutDataType=fixdt(1,16,0)  OutScaling=[]  RndMeth=Zero
  2 : Outport  OutDataType=fixdt(1,16,0)  OutScaling=[]
  wires:
  1/1 -> Gain_1/1
  Gain_1/1 -> 2/1

== system FullEKF_2007a/INS/Attitude update/Stage2/Subsystem/a31/product ==
  1 : Inport  OutDataType=fixdt(1,16,0)  OutScaling=[]
  2 : Inport  Port=2  OutDataType=fixdt(1,16,0)  OutScaling=[]
  Product_1 : Product  OutDataType=fixdt(1,16,0)  OutScaling=[]  RndMeth=Zero  InputSameDT=on
  1000 : Outport  OutDataType=fixdt(1,16,0)  OutScaling=[]
  wires:
  Product_1/1 -> 1000/1
  1/1 -> Product_1/1
  2/1 -> Product_1/2

== system FullEKF_2007a/INS/Attitude update/Stage2/Subsystem/a31/product1 ==
  1 : Inport  OutDataType=fixdt(1,16,0)  OutScaling=[]
  2 : Inport  Port=2  OutDataType=fixdt(1,16,0)  OutScaling=[]
  Product_1 : Product  OutDataType=fixdt(1,16,0)  OutScaling=[]  RndMeth=Zero  InputSameDT=on
  1000 : Outport  OutDataType=fixdt(1,16,0)  OutScaling=[]
  wires:
  Product_1/1 -> 1000/1
  1/1 -> Product_1/1
  2/1 -> Product_1/2

== system FullEKF_2007a/INS/Attitude update/Stage2/Subsystem/a31/sum ==
  1 : Inport  OutDataType=fixdt(1,16,0)  OutScaling=[]
  2 : Inport  Port=2  OutDataType=fixdt(1,16,0)  OutScaling=[]
  Sum_1 : Sum  OutDataType=fixdt(1,16,0)  OutScaling=[]  RndMeth=Zero  InputSameDT=on
  1000 : Outport  OutDataType=fixdt(1,16,0)  OutScaling=[]
  wires:
  Sum_1/1 -> 1000/1
  1/1 -> Sum_1/1
  2/1 -> Sum_1/2

== system FullEKF_2007a/INS/Attitude update/Stage2/Subsystem/a32/BorderBottom ==

== system FullEKF_2007a/INS/Attitude update/Stage2/Subsystem/a32/BorderLeft ==

== system FullEKF_2007a/INS/Attitude update/Stage2/Subsystem/a32/BorderRight ==

== system FullEKF_2007a/INS/Attitude update/Stage2/Subsystem/a32/BorderTop ==

== system FullEKF_2007a/INS/Attitude update/Stage2/Subsystem/a32/Subsystem Revision ==

== system FullEKF_2007a/INS/Attitude update/Stage2/Subsystem/a32/deMux ==
  Dmx : Inport  OutDataType=fixdt(1,16,0)  OutScaling=[]
  999 : Demux
  1 : Outport  OutDataType=fixdt(1,16,0)  OutScaling=[]
  2 : Outport  Port=2  OutDataType=fixdt(1,16,0)  OutScaling=[]
  3 : Outport  Port=3  OutDataType=fixdt(1,16,0)  OutScaling=[]
  4 : Outport  Port=4  OutDataType=fixdt(1,16,0)  OutScaling=[]
  wires:
  999/1 -> 1/1
  999/2 -> 2/1
  Dmx/1 -> 999/1
  999/3 -> 3/1
  999/4 -> 4/1

== system FullEKF_2007a/INS/Attitude update/Stage2/Subsystem/a32/gain ==
  1 : Inport  OutDataType=fixdt(1,16,0)  OutScaling=[]
  Gain_1 : Gain  Gain=eval(gain)  ParameterDataType=fixdt(1,16,0)  ParameterScaling=[]  OutDataType=fixdt(1,16,0)  OutScaling=[]  RndMeth=Zero
  2 : Outport  OutDataType=fixdt(1,16,0)  OutScaling=[]
  wires:
  1/1 -> Gain_1/1
  Gain_1/1 -> 2/1
